simulink model "s10_5"  (Simulink 6.6)
settings: Solver=FixedStepDiscrete  SolverMode=SingleTasking  StartTime=0.0  StopTime=t_d  MaxStep=Tc  RelTol=1e-6  AbsTol=1e-6
values from neighbouring files (symbols this model uses):
  k_s = 160    [i10_5.m]
  s = features_l(sp0)    [i10_5.m]
  Tc = 0.001    [i10_5.m]
  Ts = Tc    (= 0.001)    [i10_5.m]
  xh0 = [0; 0; 0.5; 0]    [i10_5.m]
undefined symbols (not defined in the file or in its folder): DiscIntNeverNeededParam
settings Model: Creator=luigivillani  LastModifiedBy=luigivillani  ExtModeAutoUpdateStatusClock=off
settings DataIOCC: LimitDataPoints=off  SaveOutput=off  SaveTime=off  SignalLoggingName=sigsOut
settings OptimizationCC: BooleanDataType=off
settings DebuggingCC: SignalResolutionControl=TryResolveAllWithWarning  SolverPrmCheckMsg=none  MultiTaskDSMMsg=warning  MultiTaskCondExecSysMsg=none  StrictBusMsg=None
settings HardwareCC: TargetUnknown=on
settings RTWCC: IncludeERTFirstTime=on

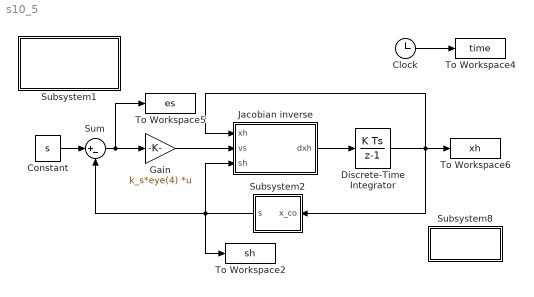
== system s10_5 ==
  Clock : Clock
      settings: Decimation=10
  Constant : Constant  Value=s  SampleTime=Tc
  Discrete-Time Integrator : DiscreteIntegrator  InitialCondition=xh0  SampleTime=Tc  ICPrevOutput=DiscIntNeverNeededParam  ICPrevScaledInput=DiscIntNeverNeededParam
  Gain : Gain  Gain=k_s*eye(4)  Multiplication=Matrix(K*u)  SampleTime=Tc
      mask Display: disp('K_s')
  Jacobian inverse : Subsystem
      mask Display: disp('inv(J_asl)vs')
  Subsystem1 : Subsystem
      settings: OpenFcn=clear all;i10_5;
      mask Display: disp('variables\n initialization')
  Subsystem2 : Subsystem  Orientation=left
      mask Display: disp('sl(xh)')
  Subsystem8 : Subsystem
      settings: OpenFcn=p10_5;
      mask Display: disp('plot')
  Sum : Sum  Inputs=|+-  SaturateOnIntegerOverflow=on
  To Workspace2 : ToWorkspace  VariableName=sh  SampleTime=Ts  SaveFormat=Array
      settings: MaxDataPoints=4001
  To Workspace4 : ToWorkspace  VariableName=time  SampleTime=Ts  SaveFormat=Array
      settings: MaxDataPoints=4001
  To Workspace5 : ToWorkspace  VariableName=es  SampleTime=Ts  SaveFormat=Array
      settings: MaxDataPoints=4001
  To Workspace6 : ToWorkspace  VariableName=xh  SampleTime=Ts  SaveFormat=Array
      settings: MaxDataPoints=4001
  wires:
  Clock/1 -> To Workspace4/1
  Discrete-Time Integrator/1 -> To Workspace6/1, Jacobian inverse/1(xh), Subsystem2/1(x_co)
  Jacobian inverse/1(dxh) -> Discrete-Time Integrator/1
  Gain/1 -> Jacobian inverse/2(vs)
  Subsystem2/1(s) -> Sum/2, To Workspace2/1, Jacobian inverse/3(sh)
  Sum/1 -> To Workspace5/1, Gain/1
  Constant/1 -> Sum/1

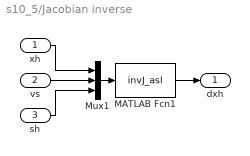
== system s10_5/Jacobian inverse ==
  xh : Inport
  vs : Inport  Port=2
  sh : Inport  Port=3
  MATLAB Fcn1 : MATLABFcn  MATLABFcn=invJ_asl  OutputDimensions=4
      mask Display: disp('inv(J_asl)')
  Mux1 : Mux  Inputs=[4,4,4]
  dxh : Outport
  wires:
  Mux1/1 -> MATLAB Fcn1/1
  xh/1 -> Mux1/1
  sh/1 -> Mux1/3
  MATLAB Fcn1/1 -> dxh/1
  vs/1 -> Mux1/2

== system s10_5/Subsystem1 ==
  note: start

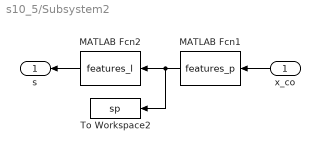
== system s10_5/Subsystem2 ==
  x_co : Inport  Orientation=left
  MATLAB Fcn1 : MATLABFcn  Orientation=left  MATLABFcn=features_p  OutputDimensions=4  SampleTime=Tc
      mask Display: disp('points')
  MATLAB Fcn2 : MATLABFcn  Orientation=left  MATLABFcn=features_l  OutputDimensions=4  SampleTime=Tc
      mask Display: disp('line')
  To Workspace2 : ToWorkspace  VariableName=sp  SampleTime=Ts  SaveFormat=Array
      settings: MaxDataPoints=4001
  s : Outport  Orientation=left
  wires:
  MATLAB Fcn1/1 -> MATLAB Fcn2/1, To Workspace2/1
  x_co/1 -> MATLAB Fcn1/1
  MATLAB Fcn2/1 -> s/1

== system s10_5/Subsystem8 ==
  note: start
